simulink model "trimtest"  (Simulink 7.7)
settings: Solver=ode45  SolverMode=SingleTasking  StartTime=0.0  StopTime=20  RelTol=1e-3  AbsTol=1e-6
StartFcn:
  | rand; global x_tr
undefined symbols (not defined in the file or in its folder): i
CloseFcn:
  | ;slview('closediagram',bdroot);
settings Model: Creator=jjbuchholz  LastModifiedBy=jjbuchholz
settings DataIOCC: LimitDataPoints=off
settings OptimizationCC: BlockReduction=off  BooleanDataType=off
settings DebuggingCC: SaveWithParameterizedLinksMsg=none  SignalResolutionControl=TryResolveAllWithWarning  SolverPrmCheckMsg=none  MultiTaskDSMMsg=warning  MultiTaskCondExecSysMsg=none  InitInArrayFormatMsg=none  StrictBusMsg=None
settings HardwareCC: TargetUnknown=on
settings RTWCC: TemplateMakefile=grt_vc.tmf  IncludeERTFirstTime=on

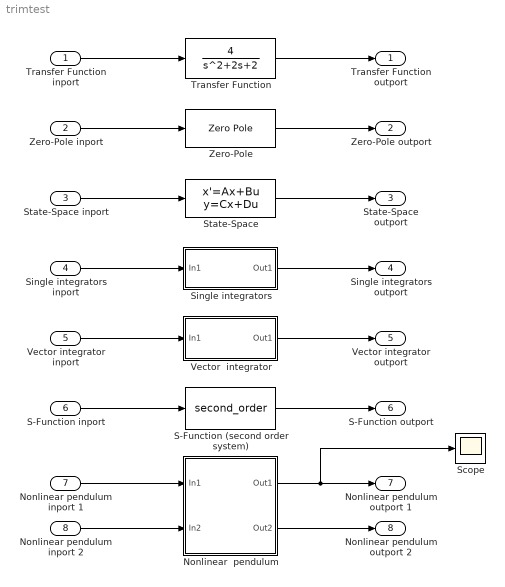
== system trimtest ==
  Transfer Function inport : Inport
  Zero-Pole inport : Inport  Port=2
  State-Space inport : Inport  Port=3
  Single integrators inport : Inport  Port=4
  Vector integrator inport : Inport  Port=5
  S-Function inport : Inport  Port=6
  Nonlinear pendulum inport 1 : Inport  Port=7
  Nonlinear pendulum inport 2 : Inport  Port=8
  Nonlinear  pendulum : Subsystem
  S-Function (second order system) : S-Function  FunctionName=second_order  EnableBusSupport=off
  Scope : Scope
      settings: TickLabels=on  YMin=0  YMax=180  DataFormat=Array
  Single integrators : Subsystem
  State-Space : StateSpace  A=[0, 1; -2, -2]  B=[0; 4]  C=[1, 0]  D=0
  Transfer Function : TransferFcn  Numerator=4  Denominator=[1, 2, 2]
  Vector  integrator : Subsystem
  Zero-Pole : ZeroPole  Zeros=[]  Poles=[-1+i; -1-i]  Gain=4
  Transfer Function outport : Outport
  Zero-Pole outport : Outport  Port=2
  State-Space outport : Outport  Port=3
  Single integrators outport : Outport  Port=4
  Vector integrator outport : Outport  Port=5
  S-Function outport : Outport  Port=6
  Nonlinear pendulum outport 1 : Outport  Port=7
  Nonlinear pendulum outport 2 : Outport  Port=8
  wires:
  Vector integrator inport/1 -> Vector  integrator/1(In1)
  S-Function inport/1 -> S-Function (second order system)/1
  Single integrators inport/1 -> Single integrators/1(In1)
  Transfer Function inport/1 -> Transfer Function/1
  Zero-Pole inport/1 -> Zero-Pole/1
  State-Space inport/1 -> State-Space/1
  Nonlinear pendulum inport 1/1 -> Nonlinear  pendulum/1(In1)
  Nonlinear pendulum inport 2/1 -> Nonlinear  pendulum/2(In2)
  Vector  integrator/1(Out1) -> Vector integrator outport/1
  Single integrators/1(Out1) -> Single integrators outport/1
  S-Function (second order system)/1 -> S-Function outport/1
  State-Space/1 -> State-Space outport/1
  Zero-Pole/1 -> Zero-Pole outport/1
  Transfer Function/1 -> Transfer Function outport/1
  Nonlinear  pendulum/2(Out2) -> Nonlinear pendulum outport 2/1
  Nonlinear  pendulum/1(Out1) -> Nonlinear pendulum outport 1/1, Scope/1

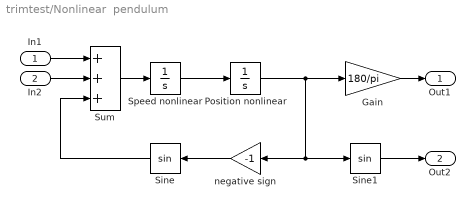
== system trimtest/Nonlinear  pendulum ==
  In1 : Inport
  In2 : Inport  Port=2
  Gain : Gain  Gain=180/pi  SaturateOnIntegerOverflow=on  OutDataTypeStr=Inherit: Same as input  ParamDataTypeStr=Inherit: Same as input
  Position nonlinear : Integrator
  Sine : Trigonometry
  Sine1 : Trigonometry
  Speed nonlinear : Integrator
  Sum : Sum  Inputs=3  SaturateOnIntegerOverflow=on  InputSameDT=on  OutDataTypeStr=Inherit: Same as first input
  negative sign : Gain  Gain=-1  SaturateOnIntegerOverflow=on  OutDataTypeStr=Inherit: Same as input  ParamDataTypeStr=Inherit: Same as input
  Out1 : Outport  InitialOutput=0
  Out2 : Outport  Port=2  InitialOutput=0
  wires:
  negative sign/1 -> Sine/1
  Speed nonlinear/1 -> Position nonlinear/1
  Position nonlinear/1 -> Gain/1, negative sign/1, Sine1/1
  Gain/1 -> Out1/1
  Sine1/1 -> Out2/1
  Sum/1 -> Speed nonlinear/1
  Sine/1 -> Sum/3
  In1/1 -> Sum/1
  In2/1 -> Sum/2

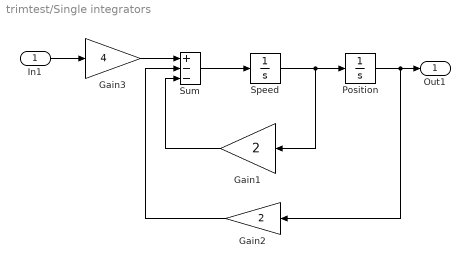
== system trimtest/Single integrators ==
  In1 : Inport
  Gain1 : Gain  Gain=2  SaturateOnIntegerOverflow=on  OutDataTypeStr=Inherit: Same as input  ParamDataTypeStr=Inherit: Same as input
  Gain2 : Gain  Gain=2  SaturateOnIntegerOverflow=on  OutDataTypeStr=Inherit: Same as input  ParamDataTypeStr=Inherit: Same as input
  Gain3 : Gain  Gain=4  SaturateOnIntegerOverflow=on  OutDataTypeStr=Inherit: Same as input  ParamDataTypeStr=Inherit: Same as input
  Position : Integrator
  Speed : Integrator
  Sum : Sum  Inputs=+--  SaturateOnIntegerOverflow=on  InputSameDT=on  OutDataTypeStr=Inherit: Same as first input
  Out1 : Outport  InitialOutput=0
  wires:
  In1/1 -> Gain3/1
  Sum/1 -> Speed/1
  Gain1/1 -> Sum/3
  Speed/1 -> Position/1, Gain1/1
  Gain2/1 -> Sum/2
  Position/1 -> Gain2/1, Out1/1
  Gain3/1 -> Sum/1

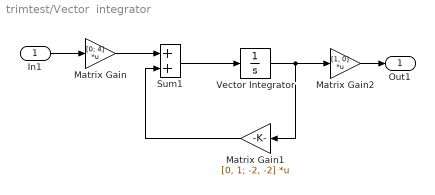
== system trimtest/Vector  integrator ==
  In1 : Inport
  Matrix Gain : Gain  Gain=[0; 4]  Multiplication=Matrix(K*u)  SaturateOnIntegerOverflow=on  OutDataTypeStr=Inherit: Same as input  ParamDataTypeStr=Inherit: Same as input
  Matrix Gain1 : Gain  Gain=[0, 1; -2, -2]  Multiplication=Matrix(K*u)  SaturateOnIntegerOverflow=on  OutDataTypeStr=Inherit: Same as input  ParamDataTypeStr=Inherit: Same as input
  Matrix Gain2 : Gain  Gain=[1, 0]  Multiplication=Matrix(K*u)  SaturateOnIntegerOverflow=on  OutDataTypeStr=Inherit: Same as input  ParamDataTypeStr=Inherit: Same as input
  Sum1 : Sum  SaturateOnIntegerOverflow=on  InputSameDT=on  OutDataTypeStr=Inherit: Same as first input
  Vector Integrator : Integrator  InitialCondition=[0 0]
  Out1 : Outport  InitialOutput=0
  wires:
  In1/1 -> Matrix Gain/1
  Sum1/1 -> Vector Integrator/1
  Matrix Gain/1 -> Sum1/1
  Vector Integrator/1 -> Matrix Gain2/1, Matrix Gain1/1
  Matrix Gain1/1 -> Sum1/2
  Matrix Gain2/1 -> Out1/1
